simulink library "dspsrcs4"  (Simulink 8.2)
settings: Solver=ode45  SolverMode=SingleTasking  StartTime=0.0  StopTime=10.0  RelTol=1e-3
undefined symbols (not defined in the file or in its folder): Low
libraries: dspmtrx3 x2, dspvision x1, dspswit3 x1, dspnetwork x1
settings Model: RequirementInfo=9  Creator=lelas  LastModifiedBy=prana  CovMetricSettings=d  ExtModeAutoUpdateStatusClock=off
settings Model: ForwardingTableString=|
  | ||__slOldName__||dspsrcs4/DSP
  | Constant||__slNewName__||dspobslib/DSP
  | Constant||__slOldName__||dspsrcs4/Constant Ramp||__slNewName__||dspsigops/Constant Ramp||__slOldName__||dspsrcs4/Triggered Signal
  | From Workspace||__slNewName__||dspsigops/Triggered Signal
  | From Workspace||__slOldName__||dspsrcs4/From Wave File||__slNewName__||dspwin32/From Wave File||__slOldName__||dspsrcs4/From Multimedia File||__slNewName__||dspvision/From Multimedia File

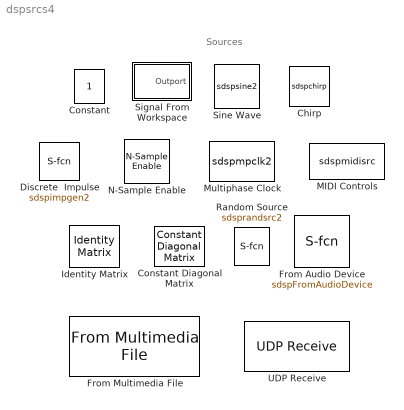
== system dspsrcs4 ==
  note: Sources
  Chirp : S-Function  FunctionName=sdspchirp  Parameters=sweep, mode, f0, f1, t1, Tsweep, phase, Ts, spf, datatype  EnableBusSupport=off  mask(Chirp){sweep=Linear, mode=Unidirectional, f0=1000, f1=4000, t1=1, Tsweep=1, phase=0, Ts=1/8000, spf=1, datatype=Double}
      mask prompts: sweep "Frequency sweep:"; mode "Sweep mode:"; f0 "Initial frequency (Hz):"; f1 "Target frequency (Hz):"; t1 "Target time (s):"; Tsweep "Sweep time (s):"; phase "Initial phase (rad):"; Ts "Sample time:"; spf "Samples per frame:"; datatype "Output data type:"
      mask help: Linear, Logarithmic, and Quadratic modes generate a swept-frequency cosine with instantaneous frequency values specified by the frequency and time parameters. The Swept cosine mode generates a swept-frequency cosine with a linear instantaneous output frequency that may differ from the one specified by the frequency and time parameters.
      mask init:
      | [t,y,txt] = dspblkchirp2('icon');
      | dspblkchirp2('param', true, sweep, f0, f1);
      mask Help: eval('blocksethelp');
      mask TypeOptions sweep: Swept cosine | Linear | Logarithmic | Quadratic
      mask TypeOptions mode: Unidirectional | Bidirectional
      mask TypeOptions datatype: Double | Single
      mask Display:
      | plot(t,y);
      | text(.2,.85,txt)
  Constant : Constant  VectorParams1D=off
  Constant Diagonal Matrix : dspmtrx3/Constant Diagonal Matrix  q=ones(1,3)  frame=off  dataType=Inherit from 'Constant(s) along diagonal'  isSigned=on  wordLen=16  udDataType=sfix(16)  fracBitsMode=Best precision  numFracBits=15
  Discrete  Impulse : S-Function  FunctionName=sdspimpgen2  Parameters=Delay, SampleTime, FrameSample, isCustomFloat, fxpIsSigned, dTypeID, fxpWordLength, fxpFracLength, [0 1]  EnableBusSupport=off  mask(Discrete Impulse){Delay=0, SampleTime=1, FrameSample=1, additionalParams=off, allowOverrides=on, dataType=double, isSigned=on, wordLen=16, udDataType=sfix(16), fracBitsMode=Best precision, numFracBits=15, OutDataTypeStr=double, LastOutDataTypeStr=double}
      mask prompts: Delay "Delay (samples):"; SampleTime "Sample time:"; FrameSample "Samples per frame:"; additionalParams "------- Show additional parameters --------"; allowOverrides "Allow overrides from DSP Fixed-Point Attributes blocks"; dataType "Output data type:"; isSigned "Signed"; wordLen "Word length:"; udDataType "User-defined data type (e.g. sfix(16), float('single')):"; fracBitsMode "Set fraction length in output to:"; numFracBits "Fraction length:"; OutDataTypeStr "Output data type:"; LastOutDataTypeStr "Last output data type string:"
      mask help: Output a discrete unit impulse. The impulse will be offset by the number of samples in the Delay parameter.
      mask init:
      | dTypeID       = 0; % nice default
      | isCustomFloat = 0; % nice default
      | fxpIsSigned   = 1; % nice default
      | fxpWordLength = 8; % nice default
      | fxpFracLength = 0; % nice default
      | dtRows = dspblkGetDiscreteImpulseDTRowInfo();
      | [dtInfo, dTypeID] = dspblkUDTMapperOutDType(gcbh, dtRows{1}, 'dataType', 1.0);
      | isCustomFloat     = dtInfo.DataTypeIsCustomFloat;
      | if ~isCustomFloat
      |     fxpIsSigned   = dtInfo.DataTypeIsSigned;
      |     fxpWordLength = dtInfo.DataTypeWordLength;
      |     fxpFracLength = dtInfo.DataTypeFracOrMantBits;
      | end
      mask Help: eval('blocksethelp');
      mask TypeOptions dataType: double | single | int8 | uint8 | int16 | uint16 | int32 | uint32 | boolean | Fixed-point | User-defined | Inherit via back propagation
      mask TypeOptions fracBitsMode: Best precision | User-defined
      mask Display:
      | % Set up rectangular boxes/data points
      | nPts = 5;
      | dist = 0.6/nPts;
      | dx   = dist/3; dy = dist/3;
      | x    = (.1:1/nPts:.9);
      | z    = zeros(size(x));
      | imp  = [0 0 .5-dy 0 0];
      | y    = [0 0 .5 0 0];
      | n = NaN; n = n(ones(size(x)));
      | xn   = [x-dx; x+dx; x+dx; x-dx; x-dx; n; x; x; n];
      | yn   = [y-dy; y-dy; y+dy; y+dy; y-dy; n; z; imp; n];
      | 
      | % Set up x-axis
      | v = x;
      | offset = dx;
      | xline=[v(1)+offset v(2)-offset NaN v(2)+offset v(4)-offset NaN ...
      |     v(4)+offset v(5)-offset];
      | yline=[0 0 NaN 0 0 NaN 0 0];
      | 
      | % Final plotting variables
      | xn=xn(:);
      | yn=yn(:);
      | x=[xn; NaN; xline'];
      | y=[yn; NaN; yline'];
      | plot(x,y)
  From Audio Device : S-Function  DialogController=dspDDGCreate  DialogControllerArgs=DataTag0  FunctionName=sdspFromAudioDevice  Parameters=deviceName, numChannels, sampleRate, deviceDatatype, autoBufferSize, bufferSize, queueDuration, frameSize, outputDatatype, defaultInputChannelMapping, inputChannelMapping  EnableBusSupport=off  mask(From Audio Device){deviceName=Default, numChannels=2, sampleRate=44100, deviceDatatype=Determine from output data type, autoBufferSize=on, bufferSize=4096, queueDuration=1.0, frameSize=1024, outputDatatype=double, defaultInputChannelMapping=on, inputChannelMapping=1}
      mask prompts: deviceName "Device name"; numChannels "Number of channels"; sampleRate "Sample rate"; deviceDatatype "Device data type"; autoBufferSize "Automatically determine buffer size"; bufferSize "Buffer size (samples)"; queueDuration "Queue duration"; frameSize "Frame size"; outputDatatype "Output data type"; defaultInputChannelMapping "Use default mapping between Device Input Channels and Data"; inputChannelMapping "Device Input Channels"
      mask help: Record sound data from your computer's audio device.
      mask init:
      | icon = dspdialog.FromAudioDevice.maskInit();
      mask Help: eval('blocksethelp');
      mask TypeOptions deviceDatatype: Determine from output data type | 8-bit integer | 16-bit integer | 24-bit integer | 32-bit float
      mask TypeOptions outputDatatype: uint8 | int16 | int32 | single | double
      mask Display:
      | patch(icon.x1, icon.y1);
      | patch(icon.x, icon.y, [1 1 1]*.5);
      | patch(icon.x2, icon.y2);
      | plot(-.4,0,1.4,2)
  From Multimedia File : dspvision/From Multimedia File  inputFilename=speech_dft.mp3  loop=on  numPlays=inf  outputStreams=Audio only  videoDataType=single  audioDataType=double  inheritSampleTime=on  userDefinedSampleTime=1/30  noAudioOutput=off  isIntensityVideo=off  fourcc=RGB  colorVideoFormat=Separate color signals  outputEOF=off  dataOrg=Column-major  audioFrameSize=1024  computeAudioFrameSize=off  outSamplingMode=Frame based
  Identity Matrix : dspmtrx3/Identity Matrix  Inherit=off  N=5  Ts=1  dataType=double  isSigned=on  wordLen=16  udDataType=sfix(16)  fracBitsMode=Best precision  numFracBits=15  OutDataTypeStr=double  LastOutDataTypeStr=double
  MIDI Controls : S-Function  FunctionName=sdspmidisrc  Parameters=UseSpecifiedControls,ControlNumbers, InitialValues, UseSpecifiedDevice, DeviceName, SyncAtStart, RawUint8  EnableBusSupport=off  mask(MIDI Controls){UseSpecifiedDevice=Default, DeviceName='', UseSpecifiedControls=Respond to any control, ControlNumbers=0, InitialValues=0, SyncAtStart=off, RawUint8=Normalized (0 - 1)}
      mask prompts: UseSpecifiedDevice "MIDI device:"; DeviceName "MIDI device name:"; UseSpecifiedControls "MIDI controls:"; ControlNumbers "MIDI control numbers:"; InitialValues "Initial values:"; SyncAtStart "Send initial values to device at start"; RawUint8 "Output mode:"
      mask help:
      | Output values from controls on a MIDI control surface.  Use a vector of control numbers to output values for multiple controls.
      |
      | Use the MATLAB midiid command to discover MIDI device names or MIDI device control numbers.
      mask Help: eval('blocksethelp');
      mask TypeOptions UseSpecifiedDevice: Default	 | Specify other
      mask Callback UseSpecifiedDevice:
      | switch 2*~isempty(strfind(get_param(gcbh,'UseSpecifiedDevice'),'pecif')) ...
      |         + ~isempty(strfind(get_param(gcbh,'UseSpecifiedControls'),'pecif'))
      |     case 0
      |         set_param(gcbh,'MaskVisibilities',{'on','off','on','off','on','on','on'});
      |     case 1
      |         set_param(gcbh,'MaskVisibilities',{'on','off','on','on','on','on','on'});
      |     case 2
      |         set_param(gcbh,'MaskVisibilities',{'on','on','on','off','on','on','on'});
      |     case 3
      |         set_param(gcbh,'MaskVisibilities',{'on','on','on','on','on','on','on'});
      | end
      mask TypeOptions UseSpecifiedControls: Respond to any control | Respond to specified controls
      mask Callback UseSpecifiedControls:
      | switch 2*~isempty(strfind(get_param(gcbh,'UseSpecifiedDevice'),'pecif')) ...
      |         + ~isempty(strfind(get_param(gcbh,'UseSpecifiedControls'),'pecif'))
      |     case 0
      |         set_param(gcbh,'MaskVisibilities',{'on','off','on','off','on','on','on'});
      |     case 1
      |         set_param(gcbh,'MaskVisibilities',{'on','off','on','on','on','on','on'});
      |     case 2
      |         set_param(gcbh,'MaskVisibilities',{'on','on','on','off','on','on','on'});
      |     case 3
      |         set_param(gcbh,'MaskVisibilities',{'on','on','on','on','on','on','on'});
      | end
      mask TypeOptions RawUint8: Normalized (0 - 1) | Raw MIDI (0 - 127)
      mask Display: disp('MIDI Controls')
  Multiphase Clock : S-Function  FunctionName=sdspmpclk2  Parameters=ClkFreq, NumPhases, ActiveLevel, DutyCycle, StartPhase,DataType  EnableBusSupport=off  mask(Multiphase Clock){ClkFreq=1, NumPhases=4, StartPhase=1, DutyCycle=3, ActiveLevel=High (1), DataType=Logical}
      mask prompts: ClkFreq "Clock frequency (Hz):"; NumPhases "Number of phases, N:"; StartPhase "Starting phase (1 to N):"; DutyCycle "Number of phase intervals over which clock is active (1 to N-1):"; ActiveLevel "Active level (polarity):"; DataType "Output data type:"
      mask help: Generate a vector of N binary signals representing the N clock phases.
      mask init:
      | NumPhasesValue = get_param(gcbh, 'NumPhases');
      | if isempty(NumPhases), s=NumPhasesValue;
      | else s=num2str(NumPhases);
      | end
      | s=[s '-Phase\nClock'];
      mask Help: eval('blocksethelp');
      mask TypeOptions ActiveLevel: High (1) | Low (0)
      mask TypeOptions DataType: Logical | Boolean
      mask Display: disp(s)
  N-Sample Enable : dspswit3/N-Sample Enable  N=8  ActiveLevel=Low (0)  reset=off  TriggerType=Rising edge  Ts=1  DataType=Logical
  Random Source : S-Function  FunctionName=sdsprandsrc2  Parameters=SrcType,NormMethod,CltLength,MinVal,MaxVal,MeanVal,VarVal,RepMode,rawSeed,transformSeed,IsInherit,SampMode,SampTime,SampFrame,DataType,OutComplex  EnableBusSupport=off  mask(Random Source){SrcType=Uniform, NormMethod=Ziggurat, CltLength=12, MinVal=0, MaxVal=1, MeanVal=0, VarVal=1, RepMode=Not repeatable, rawSeed=1, IsInherit=off, SampMode=Discrete, SampTime=1, SampFrame=1, DataType=Double, OutComplex=Real}
      mask prompts: SrcType "Source type:"; NormMethod "Method:"; CltLength "Number of uniform values to sum:"; MinVal "Minimum:"; MaxVal "Maximum:"; MeanVal "Mean:"; VarVal "Variance:"; RepMode "Repeatability:"; rawSeed "Initial seed:"; IsInherit "Inherit output port attributes"; SampMode "Sample mode:"; SampTime "Sample time:"; SampFrame "Samples per frame:"; DataType "Output data type:"; OutComplex "Complexity:"
      mask help: Output a random signal with uniform or Gaussian (normal) distribution. Set output repeatability to Nonrepeatable (block randomly selects initial seed every time simulation starts), Repeatable (block randomly selects initial seed once and uses it every time simulation starts), or Specify seed (block uses specified initial seed every time simulation starts, producing repeatable output).
      mask init:
      | [x,y]=dspblkrandsrc2('icon');
      | if RepMode == 1
      | 	transformSeed=[];
      | else
      | 	transformSeed=eval(dspblkrandsrc2('seed'),'rawSeed');
      | end
      | if IsInherit
      |     set_param(gcb,'Diagnostics','AllowInheritedTsInSrc');
      | else
      |     set_param(gcb,'Diagnostics','');
      | end
      mask Help: eval('blocksethelp');
      mask TypeOptions SrcType: Uniform | Gaussian
      mask Callback SrcType: dspblkrandsrc2;
      mask TypeOptions NormMethod: Ziggurat | Sum of uniform values
      mask Callback NormMethod: dspblkrandsrc2;
      mask TypeOptions RepMode: Specify seed | Repeatable | Not repeatable
      mask Callback RepMode: dspblkrandsrc2;
      mask Callback IsInherit: dspblkrandsrc2;
      mask TypeOptions SampMode: Discrete | Continuous
      mask Callback SampMode: dspblkrandsrc2;
      mask TypeOptions DataType: Double | Single
      mask TypeOptions OutComplex: Real | Complex
      mask Display: plot(x,y);
  Signal From Workspace : Subsystem  mask(Signal From Workspace){X=1:10, Ts=1, nsamps=1, OutputAfterFinalValue=Setting to zero, ignoreOrWarnInputAndFrameLengths=off}
      mask prompts: X "Signal:"; Ts "Sample time:"; nsamps "Samples per frame:"; OutputAfterFinalValue "Form output after final data value by:"; ignoreOrWarnInputAndFrameLengths "Warn when frame size does not evenly divide input length"
      mask help:
      | Output signal samples obtained from the MATLAB workspace at successive sample times.  A signal matrix is interpreted as having one channel per column.  Signal columns may be buffered into frames by specifying a number of samples per frame greater than 1.
      |
      | An M x N x P signal array outputs M x N matrices at successive sample times.  The samples per frame must be equal to 1 for three-dimensional signal arrays.
      mask init:
      | dispX = get_param(gcbh, 'X');
      | [s,Ts] = dspblksfw2('init', X,Ts,nsamps);
      mask Help: eval('blocksethelp');
      mask TypeOptions OutputAfterFinalValue: Setting to zero | Holding final value | Cyclic repetition
      mask Callback OutputAfterFinalValue: dspblksfw2
      mask Display: disp(dispX)
  Sine Wave : S-Function  FunctionName=sdspsine2  Parameters=Amplitude, Frequency, Phase, SampleMode, OutComplex, CompMethod, SampleTime, SamplesPerFrame, ResetState, TableSize, isCustomFloat, fxpIsSigned, dTypeID, fxpWordLength, fxpFracLength  EnableBusSupport=off  mask(Sine Wave){Amplitude=1, Frequency=100, Phase=0, SampleMode=Discrete, OutComplex=Real, CompMethod=Trigonometric fcn, TableSize=Speed, SampleTime=1/1000, SamplesPerFrame=1, ResetState=Restart at time zero, additionalParams=off, allowOverrides=on, dataType=double, wordLen=16, udDataType=sfix(16), fracBitsMode=Best precision, numFracBits=15, OutDataTypeStr=double, LastOutDataTypeStr=double}
      mask prompts: Frequency "Frequency (Hz):"; Phase "Phase offset (rad):"; SampleMode "Sample mode:"; OutComplex "Output complexity:"; CompMethod "Computation method:"; TableSize "Optimize table for:"; SampleTime "Sample time:"; SamplesPerFrame "Samples per frame:"; ResetState "Resetting states when re-enabled:"; additionalParams "------- Show additional parameters --------"; allowOverrides "Allow overrides from DSP Fixed-Point Attributes blocks"; dataType "Output data type:"; wordLen "Word length:"; udDataType "User-defined data type (e.g. sfix(16), float('single')):"; fracBitsMode "Set fraction length in output to:"; numFracBits "Fraction length:"; OutDataTypeStr "Output data type:"; LastOutDataTypeStr "Last output data type string:"
      mask help: Output samples of a sinusoid. To generate more than one sinusoid simultaneously, enter a vector of values for the Amplitude, Frequency, and Phase offset parameters.
      mask init:
      | dType = dataType; % for obsolete library block backward compatibility
      | dTypeID       = 0; % nice default
      | isCustomFloat = 0; % nice default
      | fxpIsSigned   = 1; % nice default
      | fxpWordLength = 8; % nice default
      | fxpFracLength = 0; % nice default
      | dtRows = dspblkGetSineWaveDTRowInfo();
      | [dtInfo, dTypeID] = dspblkUDTMapperOutDType(gcbh, dtRows{1}, 'dataType', abs(Amplitude));
      | isCustomFloat     = dtInfo.DataTypeIsCustomFloat;
      | if ~isCustomFloat
      |     fxpIsSigned   = dtInfo.DataTypeIsSigned;
      |     fxpWordLength = dtInfo.DataTypeWordLength;
      |     fxpFracLength = dtInfo.DataTypeFracOrMantBits;
      | end
      mask Help: eval('blocksethelp');
      mask TypeOptions SampleMode: Discrete | Continuous
      mask Callback SampleMode: dspblksine;
      mask TypeOptions OutComplex: Real | Complex
      mask TypeOptions CompMethod: Trigonometric fcn | Table lookup | Differential
      mask Callback CompMethod: dspblksine;
      mask TypeOptions TableSize: Speed | Memory
      mask TypeOptions ResetState: Restart at time zero | Catch up to simulation time
      mask TypeOptions dataType: double | single | Fixed-point | User-defined | Inherit via back propagation
      mask TypeOptions fracBitsMode: Best precision | User-defined
      mask Display:
      | if isequal(SampleMode,1)
      |     % Discrete
      |     dx=pi/5;
      |     x=(0:dx:2*pi)';
      |     y=sin(x);
      |     [x,y]=stairs(x,y);
      | else
      |     % Continuous
      |     dx=pi/22;
      |     x=(0:dx:2*pi)';
      |     y=sin(x);
      | end
      | x=[x;NaN;0; 0;NaN;0;2*pi];
      | y=[y;NaN;1;-1;NaN;0;0];
      | plot(x,y)
      | text(3.25,.75,'DSP');
  UDP Receive : dspnetwork/UDP Receive  localURL='0.0.0.0'  localPort=25000  remoteURL='0.0.0.0'  remotePort=-1  recvBufferSize=8192  dims=255  signalDatatype=uint8  isVarSize=on  showBlockingTime=off  blockingTime=0  sampletime=1

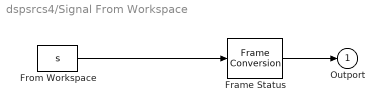
== system dspsrcs4/Signal From Workspace ==
  Frame Status : FrameConversion  OutFrame=Sample-based
  From Workspace : FromWorkspace  VariableName=s  SampleTime=Ts  Interpolate=off  OutputAfterFinalValue=Setting to zero
  Outport : Outport  InitialOutput=0
  wires:
  From Workspace/1 -> Frame Status/1
  Frame Status/1 -> Outport/1
